simulink model "phi1"  (Simulink 7.9)
settings: Solver=ode45  StartTime=0.0  StopTime=10.0  RelTol=1e-3
values from neighbouring files (symbols this model uses):
  b = 0.05    [parametrosLinealizacion.m]
  g = 9.81    [parametrosLinealizacion.m]
  I = 0.0138    [parametrosLinealizacion.m]
  M = 0.768    [parametrosLinealizacion.m]
  m = 0.104    [parametrosLinealizacion.m]
undefined symbols (not defined in the file or in its folder): ml, ml2
settings Model: Creator=root  LastModifiedBy=root

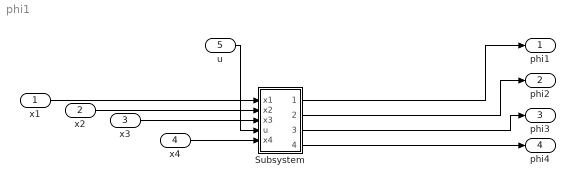
== system phi1 ==
  x1 : Inport
  x2 : Inport  Port=2
  x3 : Inport  Port=3
  x4 : Inport  Port=4
  u : Inport  Port=5
  Subsystem : Subsystem
  phi1 : Outport
  phi2 : Outport  Port=2
  phi3 : Outport  Port=3
  phi4 : Outport  Port=4
  wires:
  x1/1 -> Subsystem/1(x1)
  x2/1 -> Subsystem/2(x2)
  Subsystem/1(phi1) -> phi1/1
  Subsystem/2(phi2) -> phi2/1
  x3/1 -> Subsystem/3(x3)
  u/1 -> Subsystem/4(u)
  Subsystem/3(phi3) -> phi3/1
  Subsystem/4(phi4) -> phi4/1
  x4/1 -> Subsystem/5(x4)

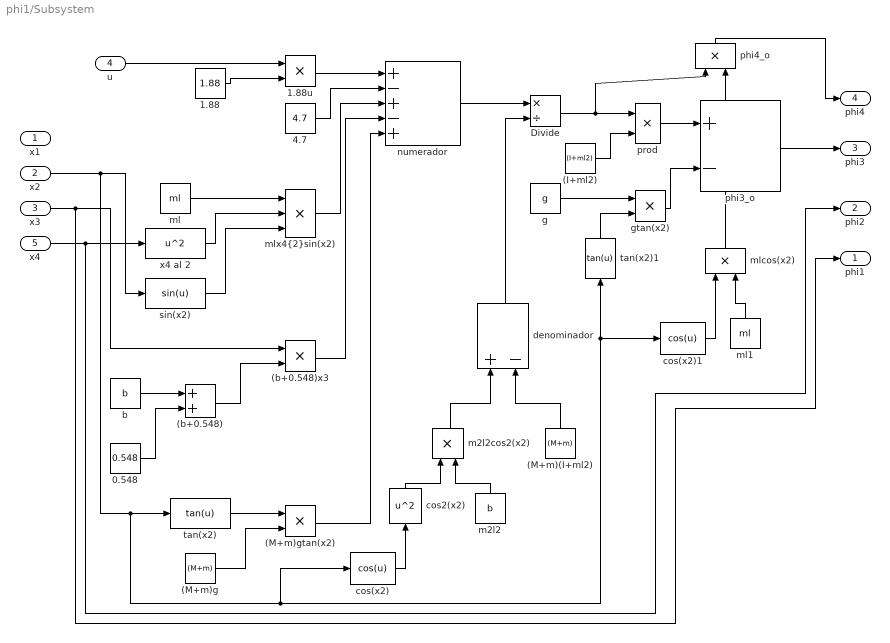
== system phi1/Subsystem ==
  x1 : Inport
  x2 : Inport  Port=2
  x3 : Inport  Port=3
  u : Inport  Port=4
  x4 : Inport  Port=5
  (I+ml2) : Constant  Value=(I+ml2)
  (M+m)(I+ml2) : Constant  Value=(M+m)
  (M+m)g : Constant  Value=(M+m)
  (M+m)gtan(x2) : Product  RndMeth=Zero
  (b+0.548) : Sum
  (b+0.548)x3 : Product  RndMeth=Zero
  0.548 : Constant  Value=0.548
  1.88 : Constant  Value=1.88
  1.88u : Product  RndMeth=Zero
  4.7 : Constant  Value=4.7
  Divide : Product  Inputs=*/
  b : Constant  Value=b
  cos(x2) : Fcn  Expr=cos(u)  SampleTime=0.1
  cos(x2)1 : Fcn  Expr=cos(u)  SampleTime=0.1
  cos2(x2) : Fcn  Expr=u^2  SampleTime=0.1
  denominador : Sum  Inputs=+-
  g : Constant  Value=g
  gtan(x2) : Product  RndMeth=Zero
  m2l2 : Constant  Value=b
  m2l2cos2(x2) : Product  RndMeth=Zero
  ml : Constant  Value=ml
  ml1 : Constant  Value=ml
  mlcos(x2) : Product  RndMeth=Zero
  "mlx4{2}sin(x2)" : Product  Inputs=3  RndMeth=Zero
  numerador : Sum  Inputs=+-+-+
  phi3_o : Sum  Inputs=+-
  phi4_o : Product  RndMeth=Zero
  prod : Product  RndMeth=Zero
  sin(x2) : Fcn  Expr=sin(u)  SampleTime=0.1
  tan(x2) : Fcn  Expr=tan(u)  SampleTime=0.1
  tan(x2)1 : Fcn  Expr=tan(u)  SampleTime=0.1
  x4 al 2 : Fcn  Expr=u^2  SampleTime=0.1
  phi1 : Outport
  phi2 : Outport  Port=2
  phi3 : Outport  Port=3
  phi4 : Outport  Port=4
  wires:
  1.88/1 -> 1.88u/2
  u/1 -> 1.88u/1
  1.88u/1 -> numerador/1
  4.7/1 -> numerador/2
  ml/1 -> "mlx4{2}sin(x2)"/1
  sin(x2)/1 -> "mlx4{2}sin(x2)"/3
  x4 al 2/1 -> "mlx4{2}sin(x2)"/2
  x4/1 -> x4 al 2/1, phi2/1
  x2/1 -> sin(x2)/1, tan(x2)/1, cos(x2)/1, tan(x2)1/1, cos(x2)1/1
  "mlx4{2}sin(x2)"/1 -> numerador/3
  (b+0.548)x3/1 -> numerador/4
  x3/1 -> (b+0.548)x3/1, phi1/1
  (b+0.548)/1 -> (b+0.548)x3/2
  b/1 -> (b+0.548)/1
  0.548/1 -> (b+0.548)/2
  (M+m)gtan(x2)/1 -> numerador/5
  tan(x2)/1 -> (M+m)gtan(x2)/1
  (M+m)g/1 -> (M+m)gtan(x2)/2
  (M+m)(I+ml2)/1 -> denominador/2
  m2l2cos2(x2)/1 -> denominador/1
  cos2(x2)/1 -> m2l2cos2(x2)/1
  m2l2/1 -> m2l2cos2(x2)/2
  cos(x2)/1 -> cos2(x2)/1
  numerador/1 -> Divide/1
  denominador/1 -> Divide/2
  Divide/1 -> prod/1, phi4_o/1
  (I+ml2)/1 -> prod/2
  prod/1 -> phi3_o/1
  gtan(x2)/1 -> phi3_o/2
  g/1 -> gtan(x2)/1
  tan(x2)1/1 -> gtan(x2)/2
  mlcos(x2)/1 -> phi4_o/2
  ml1/1 -> mlcos(x2)/2
  cos(x2)1/1 -> mlcos(x2)/1
  phi3_o/1 -> phi3/1
  phi4_o/1 -> phi4/1
